simulink model "sl_jspace"  (Simulink 8.5)
settings: Solver=ode45  StartTime=0.0  StopTime=10.0  RelTol=1e-3
libraries: roblocks x4, simulink x1
settings Model: Creator=pic  LastModifiedBy=XYD  ExtModeTrigMode=oneshot  ExtModeArmWhenConnect=off  ExtModeAutoUpdateStatusClock=off
settings DataIOCC: LimitDataPoints=off  SignalLoggingName=sigsOut
settings OptimizationCC: BlockReduction=off  BooleanDataType=off
settings DebuggingCC: SaveWithParameterizedLinksMsg=none  SignalResolutionControl=TryResolveAllWithWarning  MultiTaskDSMMsg=warning  MultiTaskCondExecSysMsg=none  FcnCallInpInsideContextMsg=UseLocalSettings
settings HardwareCC: TargetUnknown=on

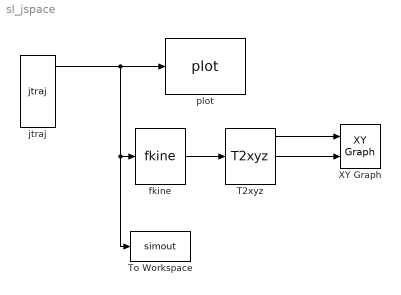
== system sl_jspace ==
  T2xyz : roblocks/Transform Conversion/T2xyz
  To Workspace : ToWorkspace  VariableName=simout  SaveFormat=Timeseries  SampleTime=-1
  XY Graph : simulink/Sinks/XY Graph  xmin=-1  xmax=1  ymin=-1  ymax=1  st=-1
  fkine : roblocks/Kinematics/fkine  robot=p560
  jtraj : roblocks/Trajectory/jtraj  q0=[0 0 0 0 0 0]  qf=[pi/4 pi/2 -pi/2 0 0 0]  tmax=10  ts=0.02
  plot : roblocks/Robot Graphics/plot  robot=p560  fps=25  holdplot=on
  wires:
  jtraj/1 -> plot/1, To Workspace/1, fkine/1
  fkine/1 -> T2xyz/1
  T2xyz/1 -> XY Graph/1
  T2xyz/2 -> XY Graph/2
